simulink model "sampleModel1566"  (R2023a)
settings: Solver=VariableStepAuto  StartTime=0.0  StopTime=10.0  RelTol=1e-3
libraries: hdlsllib x4, simulink x3
settings Model: Creator=user1  LastModifiedBy=user1

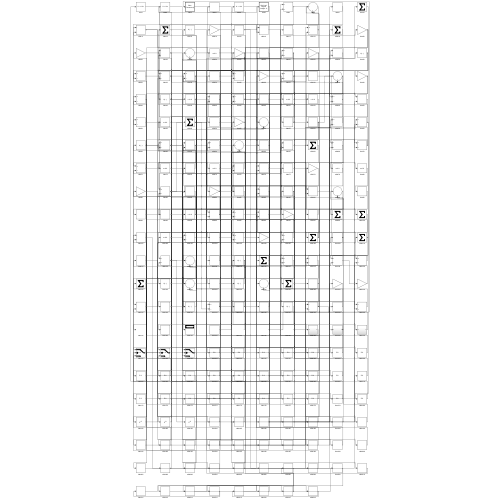
[thumbnail: Simulink's stored preview of the top-level diagram]
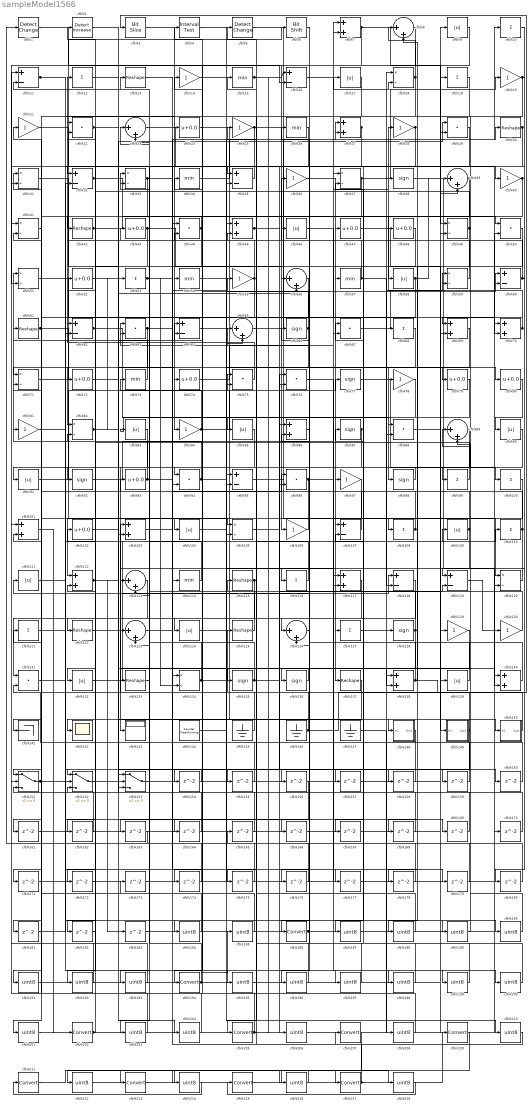
== system sampleModel1566 ==
  cfblk1 : simulink/Logic and Bit Operations/Detect Change  vinit=0  OutDataTypeStr=boolean
      settings: LibrarySourceBlock=|
      | hdlsllib/Logic and Bit
      | Operations/Detect
      | Change
  cfblk{10,12,19,53,68,99..100,108,110,116,121,127} (12 alike) : Sum  Inputs=+
  cfblk{7,27,45,69..70,86,101,103,112,117,138,140} (12 alike) : Sum
  cfblk{24,43,47..48,52,72,74,79..80,93,102} (11 alike) : Bias  Bias=0.0  SaturateOnIntegerOverflow=off
  cfblk{9,17,46,58,83,85,90..91,104,109,111,124,132,139} (14 alike) : Abs  SaturateOnIntegerOverflow=off
  cfblk{18,31,33,37,41,49,51,59,71,82,105,120,134} (13 alike) : Product  Inputs=*/  RndMeth=Zero  SaturateOnIntegerOverflow=on
  cfblk{14,20..21,25,28,36,40,55,78,81,84,97,106,129..130} (15 alike) : Gain
  cfblk{11,16,32,35,60,62,64,95,107,118..119} (11 alike) : Sum  Inputs=+-
  cfblk{8,23,39,56,65,89,113,123,126} (9 alike) : Sum  Inputs=|++
  cfblk{15,26,34,54,57,73,114} (7 alike) : MinMax
  cfblk{13,30,42,61,115,122,125,133,137} (9 alike) : Reshape
  cfblk{38,66,77,87,92,98,128,135..136} (9 alike) : Signum
  cfblk{22,29,44,50,63,67,75..76,88,94,96,131} (12 alike) : DotProduct  OutDataTypeStr=Inherit: Inherit via internal rule
  cfblk141 : Terminator
  cfblk142 : Scope
  cfblk143 : Display
  cfblk144 : hdlsllib/Sources/Counter Free-Running  NumBits=16  tsamp=-1
  cfblk145 : Ground
  cfblk146 : Ground
  cfblk147 : Ground
  cfblk148 : Subsystem
      settings: LibrarySourceBlock=|
      | hdlsllib/Ports &
      | Subsystems/Subsystem
  cfblk149 : Subsystem
      settings: LibrarySourceBlock=|
      | hdlsllib/Ports &
      | Subsystems/Subsystem
  cfblk150 : Subsystem
      settings: LibrarySourceBlock=|
      | hdlsllib/Ports &
      | Subsystems/Subsystem
  cfblk151 : Switch  SaturateOnIntegerOverflow=off  InputSameDT=off
  cfblk152 : Switch  SaturateOnIntegerOverflow=off  InputSameDT=off
  cfblk153 : Switch  SaturateOnIntegerOverflow=off  InputSameDT=off
  cfblk{154..183} (30 alike) : Delay  SampleTime=1
  cfblk{184..185,187..193,195..201,203..204,206,208,210,212,214,216,218} (25 alike) : DataTypeConversion  OutDataTypeStr=uint8  SaturateOnIntegerOverflow=off  RndMeth=Floor
  cfblk{186,194,202,205,207,209,211,213,215,217} (10 alike) : DataTypeConversion  SaturateOnIntegerOverflow=off  RndMeth=Floor
  cfblk2 : simulink/Logic and Bit Operations/Detect Increase  vinit=0.0  OutDataTypeStr=boolean
      settings: LibrarySourceBlock=|
      | hdlsllib/Logic and Bit
      | Operations/Detect
      | Increase
  cfblk3 : hdlsllib/Logic and Bit Operations/Bit Slice  lidx=7  ridx=0
  cfblk4 : hdlsllib/Logic and Bit Operations/Interval Test  IntervalClosedRight=on  uplimit=0.5  IntervalClosedLeft=on  lowlimit=-0.5  OutDataTypeStr=boolean
  cfblk5 : simulink/Logic and Bit Operations/Detect Change  vinit=0  OutDataTypeStr=boolean
      settings: LibrarySourceBlock=|
      | hdlsllib/Logic and Bit
      | Operations/Detect
      | Change
  cfblk6 : hdlsllib/Logic and Bit Operations/Bit Shift  mode=Shift Left Logical  N=0
  wires:
  cfblk119/1 -> cfblk130/1
  cfblk61/1 -> cfblk104/1, cfblk195/1
  cfblk51/1 -> cfblk137/1
  cfblk37/1 -> cfblk20/1, cfblk123/2
  cfblk9/1 -> cfblk106/1
  cfblk36/1 -> cfblk97/1
  cfblk70/1 -> cfblk28/1, cfblk69/1
  cfblk10/1 -> cfblk119/1
  cfblk24/1 -> cfblk150/1(In1)
  cfblk82/1 -> cfblk53/1, cfblk148/1(In1), cfblk158/1
  cfblk77/1 -> cfblk100/1
  cfblk94/1 -> cfblk51/1, cfblk197/1
  cfblk25/1 -> cfblk107/1, cfblk62/2, cfblk113/2
  cfblk148/1(Out1) -> cfblk83/1
  cfblk3/1 -> cfblk84/1
  cfblk149/1(Out1) -> cfblk61/1, cfblk192/1
  cfblk6/1 -> cfblk126/1
  cfblk91/1 -> cfblk77/1
  cfblk130/1 -> cfblk67/1
  cfblk42/1 -> cfblk50/1, cfblk164/1
  cfblk48/1 -> cfblk94/1
  cfblk93/1 -> cfblk55/1, cfblk81/1
  cfblk145/1 -> cfblk34/1
  cfblk66/1 -> cfblk44/2, cfblk161/1
  cfblk83/1 -> cfblk143/1
  cfblk38/1 -> cfblk140/1
  cfblk108/1 -> cfblk31/1, cfblk23/2
  cfblk115/1 -> cfblk124/1, cfblk181/1
  cfblk92/1 -> cfblk17/1
  cfblk146/1 -> cfblk103/1, cfblk69/2
  cfblk90/1 -> cfblk92/1
  cfblk5/1 -> cfblk98/1
  cfblk125/1 -> cfblk4/1
  cfblk106/1 -> cfblk105/1
  cfblk7/1 -> cfblk51/2, cfblk49/1
  cfblk102/1 -> cfblk29/1
  cfblk17/1 -> cfblk126/2
  cfblk140/1 -> cfblk26/1
  cfblk39/1 -> cfblk47/1, cfblk174/1
  cfblk71/1 -> cfblk6/1
  cfblk95/1 -> cfblk120/1
  cfblk87/1 -> cfblk132/1, cfblk153/3
  cfblk34/1 -> cfblk30/1
  cfblk75/1 -> cfblk12/1
  cfblk80/1 -> cfblk90/1
  cfblk65/1 -> cfblk10/1
  cfblk138/1 -> cfblk3/1, cfblk111/1, cfblk8/2, cfblk178/1
  cfblk22/1 -> cfblk182/1, cfblk204/1
  cfblk117/1 -> cfblk131/1
  cfblk58/1 -> cfblk39/1, cfblk157/1, cfblk175/1
  cfblk114/1 -> cfblk13/1
  cfblk68/1 -> cfblk205/1
  cfblk128/1 -> cfblk63/2, cfblk187/1
  cfblk15/1 -> cfblk16/1, cfblk206/1
  cfblk43/1 -> cfblk56/1, cfblk172/1
  cfblk40/1 -> cfblk58/1, cfblk176/1
  cfblk122/1 -> cfblk118/1
  cfblk62/1 -> cfblk114/1, cfblk56/2
  cfblk131/1 -> cfblk109/1
  cfblk153/1 -> cfblk29/2
  cfblk132/1 -> cfblk65/2
  cfblk63/1 -> cfblk82/1, cfblk169/1
  cfblk78/1 -> cfblk194/1
  cfblk96/1 -> cfblk141/1, cfblk38/1
  cfblk150/1(Out1) -> cfblk125/1
  cfblk12/1 -> cfblk74/1
  cfblk11/1 -> cfblk35/1, cfblk24/1
  cfblk97/1 -> cfblk153/2
  cfblk55/1 -> cfblk33/1, cfblk123/1
  cfblk136/1 -> cfblk133/1
  cfblk134/1 -> cfblk73/1, cfblk198/1
  cfblk85/1 -> cfblk122/1
  cfblk33/1 -> cfblk71/1, cfblk88/2
  cfblk53/1 -> cfblk88/1, cfblk134/2, cfblk159/1
  cfblk67/1 -> cfblk59/1
  cfblk99/1 -> cfblk62/1
  cfblk116/1 -> cfblk5/1
  cfblk59/1 -> cfblk22/1
  cfblk1/1 -> cfblk16/2
  cfblk107/1 -> cfblk52/1
  cfblk151/1 -> cfblk110/1, cfblk189/1
  cfblk64/1 -> cfblk117/2
  cfblk135/1 -> cfblk11/2, cfblk119/2
  cfblk144/1 -> cfblk35/2
  cfblk44/1 -> cfblk42/1, cfblk162/1
  cfblk104/1 -> cfblk27/1
  cfblk127/1 -> cfblk59/2
  cfblk23/1 -> cfblk95/1
  cfblk4/1 -> cfblk95/2
  cfblk60/1 -> cfblk36/1, cfblk180/1
  cfblk31/1 -> cfblk103/2
  cfblk30/1 -> cfblk113/1, cfblk127/1
  cfblk32/1 -> cfblk152/1, cfblk48/1
  cfblk50/1 -> cfblk79/1
  cfblk72/1 -> cfblk136/1
  cfblk137/1 -> cfblk142/1
  cfblk73/1 -> cfblk21/1
  cfblk2/1 -> cfblk105/2
  cfblk112/1 -> cfblk64/1, cfblk183/1
  cfblk18/1 -> cfblk135/1, cfblk8/1
  cfblk103/1 -> cfblk96/1
  cfblk35/1 -> cfblk32/1
  cfblk88/1 -> cfblk9/1
  cfblk8/1 -> cfblk54/1
  cfblk100/1 -> cfblk112/1
  cfblk21/1 -> cfblk70/1
  cfblk120/1 -> cfblk116/1
  cfblk123/1 -> cfblk27/2
  cfblk19/1 -> cfblk151/1
  cfblk74/1 -> cfblk7/2
  cfblk29/1 -> cfblk57/1
  cfblk54/1 -> cfblk80/1
  cfblk27/1 -> cfblk94/2, cfblk31/2, cfblk96/2
  cfblk57/1 -> cfblk118/2, cfblk45/2
  cfblk139/1 -> cfblk63/1
  cfblk124/1 -> cfblk60/1
  cfblk109/1 -> cfblk25/1, cfblk155/1
  cfblk110/1 -> cfblk46/1, cfblk193/1
  cfblk101/1 -> cfblk202/1
  cfblk133/1 -> cfblk93/1
  cfblk98/1 -> cfblk91/1
  cfblk46/1 -> cfblk70/2
  cfblk47/1 -> cfblk149/1(In1)
  cfblk49/1 -> cfblk108/1, cfblk2/1
  cfblk126/1 -> cfblk66/1
  cfblk152/1 -> cfblk75/1
  cfblk129/1 -> cfblk186/1
  cfblk45/1 -> cfblk138/2, cfblk140/2
  cfblk20/1 -> cfblk40/1, cfblk85/1, cfblk99/1
  cfblk16/1 -> cfblk18/2
  cfblk84/1 -> cfblk37/1, cfblk33/2
  cfblk28/1 -> cfblk72/1, cfblk167/1
  cfblk26/1 -> cfblk154/1
  cfblk154/1 -> cfblk152/2
  cfblk155/1 -> cfblk23/1
  cfblk118/1 -> cfblk156/1
  cfblk157/1 -> cfblk138/1
  cfblk158/1 -> cfblk65/1
  cfblk159/1 -> cfblk7/1
  cfblk105/1 -> cfblk160/1
  cfblk160/1 -> cfblk131/2
  cfblk161/1 -> cfblk117/1
  cfblk162/1 -> cfblk71/2
  cfblk79/1 -> cfblk163/1
  cfblk163/1 -> cfblk1/1
  cfblk164/1 -> cfblk82/2
  cfblk165/1 -> cfblk153/1
  cfblk81/1 -> cfblk166/1
  cfblk166/1 -> cfblk18/1
  cfblk167/1 -> cfblk39/2
  cfblk69/1 -> cfblk168/1
  cfblk168/1 -> cfblk107/2
  cfblk169/1 -> cfblk151/3
  cfblk170/1 -> cfblk37/2
  cfblk56/1 -> cfblk171/1
  cfblk171/1 -> cfblk67/2
  cfblk172/1 -> cfblk60/2
  cfblk173/1 -> cfblk75/2
  cfblk174/1 -> cfblk22/2
  cfblk175/1 -> cfblk45/1
  cfblk176/1 -> cfblk152/3
  cfblk13/1 -> cfblk177/1
  cfblk178/1 -> cfblk151/2
  cfblk111/1 -> cfblk179/1
  cfblk179/1 -> cfblk11/1
  cfblk180/1 -> cfblk64/2
  cfblk181/1 -> cfblk32/2
  cfblk182/1 -> cfblk112/2
  cfblk183/1 -> cfblk49/2
  cfblk121/1 -> cfblk184/1
  cfblk184/1 -> cfblk43/1
  cfblk185/1 -> cfblk121/1
  cfblk186/1 -> cfblk170/1, cfblk50/2
  cfblk187/1 -> cfblk129/1
  cfblk89/1 -> cfblk188/1
  cfblk188/1 -> cfblk115/1
  cfblk189/1 -> cfblk89/1
  cfblk177/1 -> cfblk190/1
  cfblk190/1 -> cfblk89/2
  cfblk41/1 -> cfblk191/1
  cfblk191/1 -> cfblk139/1
  cfblk192/1 -> cfblk41/1
  cfblk193/1 -> cfblk41/2
  cfblk194/1 -> cfblk185/1, cfblk173/1, cfblk128/1
  cfblk195/1 -> cfblk78/1
  cfblk86/1 -> cfblk196/1
  cfblk196/1 -> cfblk165/1
  cfblk197/1 -> cfblk86/1
  cfblk198/1 -> cfblk86/2
  cfblk76/1 -> cfblk199/1
  cfblk199/1 -> cfblk87/1
  cfblk52/1 -> cfblk200/1
  cfblk200/1 -> cfblk76/1
  cfblk113/1 -> cfblk201/1
  cfblk201/1 -> cfblk76/2
  cfblk202/1 -> cfblk102/1, cfblk19/1
  cfblk156/1 -> cfblk203/1
  cfblk203/1 -> cfblk101/1
  cfblk204/1 -> cfblk101/2
  cfblk205/1 -> cfblk44/1, cfblk120/2
  cfblk206/1 -> cfblk68/1
  cfblk147/1 -> cfblk208/1
  cfblk208/1 -> cfblk14/1
  cfblk14/1 -> cfblk210/1
  cfblk210/1 -> cfblk207/1
  cfblk207/1 -> cfblk212/1
  cfblk212/1 -> cfblk209/1
  cfblk209/1 -> cfblk214/1
  cfblk214/1 -> cfblk211/1
  cfblk215/1 -> cfblk217/1
  cfblk211/1 -> cfblk216/1
  cfblk216/1 -> cfblk213/1
  cfblk217/1 -> cfblk15/1, cfblk134/1
  cfblk213/1 -> cfblk218/1
  cfblk218/1 -> cfblk215/1

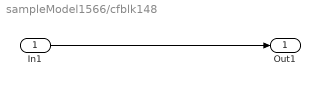
== system sampleModel1566/cfblk148 ==
  In1 : Inport
  Out1 : Outport
  wires:
  In1/1 -> Out1/1

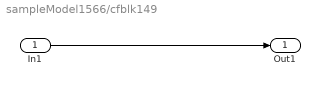
== system sampleModel1566/cfblk149 ==
  In1 : Inport
  Out1 : Outport
  wires:
  In1/1 -> Out1/1

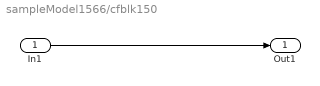
== system sampleModel1566/cfblk150 ==
  In1 : Inport
  Out1 : Outport
  wires:
  In1/1 -> Out1/1
